simulink library "TxHL_to_Enx_PWMx"  (R2014b)
settings: Solver=ode45  StartTime=0.0  StopTime=10.0  RelTol=1e-3
settings Model: Creator=vda2sh  LastModifiedBy=vda2sh

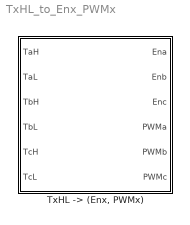
== system TxHL_to_Enx_PWMx ==
  "TxHL -> (Enx, PWMx)" : Subsystem
      mask help: This block computes the `Enx` and `PWMx` signals from the single transistor control signals `TxH` respectively `TxL`, with x in {a, b, c}.
      mask Help: Block with beta-status, actual no documentation.
      mask Display:
      | text(0.5, 0.15, 'beta')
      | port_label('input',1,'TaH [-]')
      | port_label('input',2,'TaL [-]')
      | port_label('input',3,'TbH [-]')
      | port_label('input',4,'TbL [-]')
      | port_label('input',5,'TcH [-]')
      | port_label('input',6,'TcL [-]')
      | port_label('output',1,'Ena [-]')
      | port_label('output',2,'Enb [-]')
      | port_label('output',3,'Enc [-]')
      | port_label('output',4,'PWMa [-]')
      | port_label('output',5,'PWMb [-]')
      | port_label('output',6,'PWMc [-]')

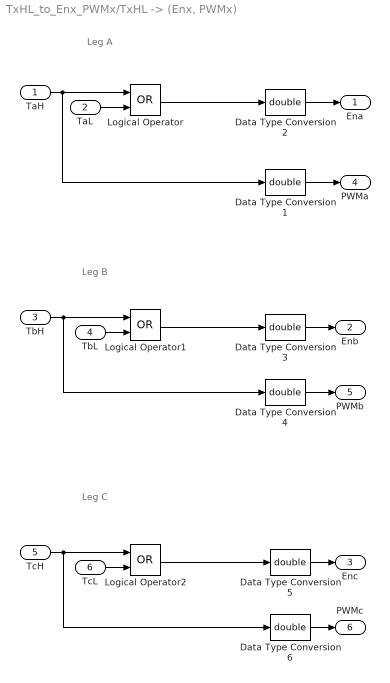
== system TxHL_to_Enx_PWMx/TxHL -> (Enx, PWMx) ==
  note: Leg A
  note: Leg B
  note: Leg C
  TaH : Inport
  TaL : Inport  Port=2
  TbH : Inport  Port=3
  TbL : Inport  Port=4
  TcH : Inport  Port=5
  TcL : Inport  Port=6
  Data Type Conversion{1..6} (6 alike) : DataTypeConversion  OutDataTypeStr=double
  Logical Operator : Logic  Operator=OR  AllPortsSameDT=off  OutDataTypeStr=boolean
  Logical Operator1 : Logic  Operator=OR  AllPortsSameDT=off  OutDataTypeStr=boolean
  Logical Operator2 : Logic  Operator=OR  AllPortsSameDT=off  OutDataTypeStr=boolean
  Ena : Outport
  Enb : Outport  Port=2
  Enc : Outport  Port=3
  PWMa : Outport  Port=4
  PWMb : Outport  Port=5
  PWMc : Outport  Port=6
  wires:
  Logical Operator/1 -> Data Type Conversion2/1
  TaL/1 -> Logical Operator/2
  Logical Operator1/1 -> Data Type Conversion3/1
  TbL/1 -> Logical Operator1/2
  TbH/1 -> Data Type Conversion4/1, Logical Operator1/1
  Logical Operator2/1 -> Data Type Conversion5/1
  TcL/1 -> Logical Operator2/2
  TcH/1 -> Data Type Conversion6/1, Logical Operator2/1
  TaH/1 -> Data Type Conversion1/1, Logical Operator/1
  Data Type Conversion2/1 -> Ena/1
  Data Type Conversion1/1 -> PWMa/1
  Data Type Conversion3/1 -> Enb/1
  Data Type Conversion4/1 -> PWMb/1
  Data Type Conversion5/1 -> Enc/1
  Data Type Conversion6/1 -> PWMc/1
